simulink model "basic_robot_motion_sim"  (R2025b)
settings: Solver=ode4  StartTime=0.0  StopTime=20  FixedStep=0.1  RelTol=1e-3
values from neighbouring files (symbols this model uses):
  dt = 0.05    [basic_robot_motion_sim_plot.m]
  omega0 = 90    [basic_robot_motion_sim_plot.m]
  v0 = 10    [basic_robot_motion_sim_plot.m]
libraries: simulink_extras x1
settings Model: PacingRate=0.500000  Creator=adity  LastModifiedBy=adity
settings OptimizationCC: BlockReduction=off  DefaultParameterBehavior=Inlined  BufferReuse=off

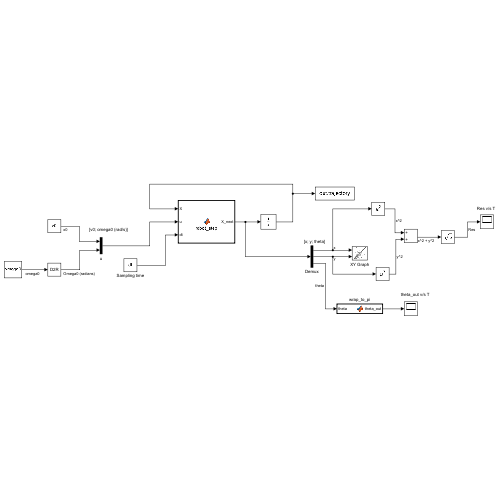
[thumbnail: Simulink's stored preview of the top-level diagram]
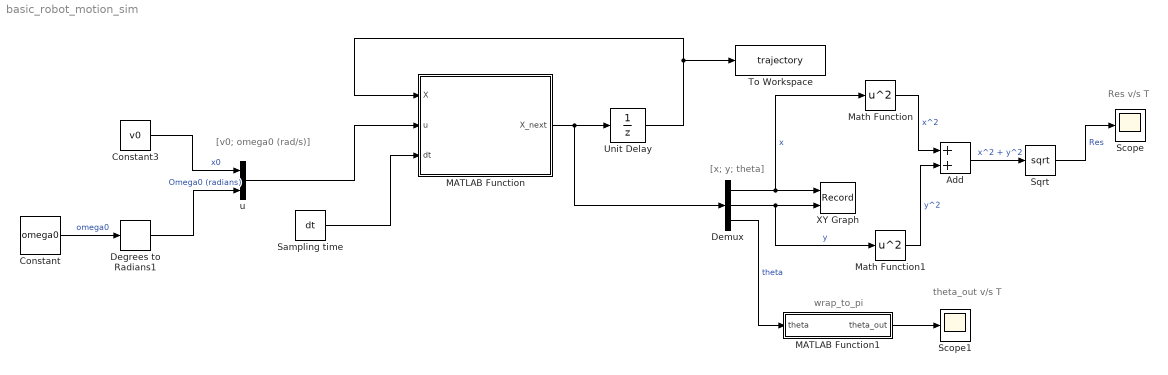
== system basic_robot_motion_sim ==
  note: wrap_to_pi
  note: theta_out v/s T
  note: [x; y; theta]
  note: [v0; omega0 (rad/s)]
  note: Res v/s T
  Add : Sum
  Constant : Constant  Value=omega0
  Constant3 : Constant  Value=v0
  Degrees to Radians1 : simulink_extras/Transformations/Degrees to Radians
  Demux : Demux  Outputs=3
  MATLAB Function : MATLAB Function  TreatAsAtomicUnit=on
  MATLAB Function1 : MATLAB Function  TreatAsAtomicUnit=on
  Math Function : Math  Operator=square
  Math Function1 : Math  Operator=square
  Sampling time : Constant  Value=dt
  Scope : Scope
      settings: ActiveDisplayYMinimum=-17.095587503028128  ActiveDisplayYMaximum=15.482305032520726
  Scope1 : Scope
      settings: ActiveDisplayYMinimum=-3.838633523605028  ActiveDisplayYMaximum=3.9171733399447732
  Sqrt : Sqrt
  To Workspace : ToWorkspace  VariableName=trajectory  SaveFormat=Timeseries  SampleTime=-1
  Unit Delay : UnitDelay  InitialCondition=[0;0;0]  SampleTime=-1  HasFrameUpgradeWarning=on
  XY Graph : Record  NumPorts=2.0  FileSettingsInternal="{\"entries\":[{\"content\":{\"excelSettings\":{\"content\":{},\"type\":\"Streamout.ExcelSettings\"},\"parquetSettings\":{\"content\":{},\"type\":\"Streamout.ParquetSettings\"}},\"type\":\"Streamout.FileSettingStorage\",\"uuid\":\"\"}],\"packageUris\":[\"http:\\/\\/schema.mathworks.com\\/mf0\\/streamout_blocks\\/R2020a\"],\"version\":\"1.0\"}"  FrameSettings=[0, 0]  Layout=[1 1]  SignalsInternal="{\"entries\":[{\"content\":{\"signals\":[{\"content\":{\"blockPath\":[],\"dimensions\":[1,1],\"domain\":\"\",\"lineColor\":\"#a2142f\",\"plots\":[ 1 ],\"port\":1,\"sid\":[\"\"],\"signalID\":1,\"signalName\":\"x\"},\"type\":\"RecordBlkView.Signal\",\"uuid\":\"\"},{\"content\":{\"blockPath\":[],\"dimensions\":[1,1],\"domain\":\"\",\"lineColor\":\"#139fff\",\"plots\":[ 1 ],\"port\":2,\"sid\":[\"\"],\"signalID\":2,\"signalName\":\"y\"},\"type\":\"RecordBlkView.Signal\",\"uuid\":\"\"}]},\"type\":\"RecordBlkView.InputSignals\",\"uuid\":\"\"}],\"packageUris\":[\"http:\\/\\/schema.mathworks.com\\/mf0\\/streamout_blocks\\/R2020a\"],\"version\":\"1.0\"}"  VisualizationBindings="{\"xyplotplugin\":{\"info\":[{\"series\":[{\"bindingParametersList\":[{\"parameter\":\"X-Axis\",\"signalID\":1,\"signalName\":\"x\"},{\"parameter\":\"Y-Axis\",\"signalID\":2,\"signalName\":\"y\"}],\"seriesID\":0}],\"subplotID\":1}]}}"  CompatibilityTag=XY
  u : Mux  Inputs=2
  wires:
  Constant/1 -> Degrees to Radians1/1  "omega0"
  Constant3/1 -> u/1  "x0"
  Degrees to Radians1/1 -> u/2  "Omega0 (radians)"
  u/1 -> MATLAB Function/2(u)
  Sampling time/1 -> MATLAB Function/3(dt)
  MATLAB Function/1(X_next) -> Demux/1, Unit Delay/1
  Unit Delay/1 -> To Workspace/1, MATLAB Function/1(X)
  Demux/1 -> XY Graph/1, Math Function/1  "x"
  Demux/2 -> XY Graph/2, Math Function1/1  "y"
  Math Function1/1 -> Add/2  "y^2"
  Math Function/1 -> Add/1  "x^2"
  Add/1 -> Sqrt/1  "x^2 + y^2"
  Sqrt/1 -> Scope/1  "Res"
  Demux/3 -> MATLAB Function1/1(theta)  "theta"
  MATLAB Function1/1(theta_out) -> Scope1/1

== matlab function basic_robot_motion_sim/MATLAB Function ==
  data: X input; u input; X_next output; dt input
function X_next = robot_step(X, u, dt)

    %X : Current Robot State [x ; y ; theta]
    %u : Control Input [v ; Omega]

    %Extracing current positional state
    x = X(1);
    y = X(2);
    theta = X(3);
    

    %Extracting current linear and angular speed
    v = u(1);
    omega = u(2);
    
    
    %Calculating next state
    x_next = x + v*cos(theta)*dt;
    y_next = y + v*sin(theta)*dt;
    theta_next = wrapToPi(theta + omega*dt);

    %Storing new position values
    X_next = [x_next; y_next; theta_next];

    
end

== matlab function basic_robot_motion_sim/MATLAB Function1 ==
  data: theta input; theta_out output
function theta_out = wrap_to_pi(theta)

theta_out = atan2(sin(theta),cos(theta));

end
